simulink model "ptest3sim2"  (Simulink 6.3)
settings: Solver=FixedStepDiscrete  SolverMode=SingleTasking  StartTime=0.0  StopTime=999999  MaxStep=10  RelTol=1e-3  AbsTol=1e-6
settings Model: Creator=munlock -all d:\work\myr12\toolbox\fuzzy\fuzzy\mfedit.m  LastModifiedBy=mbharadw  ExtModeTrigMode=oneshot  ExtModeArmWhenConnect=off  StrictBusMsg=None
settings DataIOCC: LimitDataPoints=off  SaveOutput=off  SaveTime=off
settings OptimizationCC: BooleanDataType=off
settings DebuggingCC: SolverPrmCheckMsg=none
settings HardwareCC: TargetUnknown=on
settings RTWCC: TemplateMakefile=grt_vc.tmf

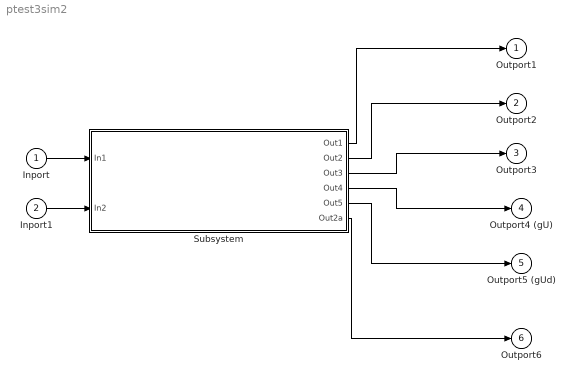
== system ptest3sim2 ==
  Inport : Inport  PortDimensions=1
  Inport1 : Inport  Port=2  PortDimensions=1
  Subsystem : Subsystem  mask{yd_init=, y_init=, ud_init=, u_init=, mint=, maxt=, minp=, maxp=, Ts=, S1=, Nu=, Normalize=, Nj=, Ni=, LW2_1=, LW1_2=, IW_gU=, IW=, B2=, B1=}
  Outport1 : Outport
  Outport2 : Outport  Port=2
  Outport3 : Outport  Port=3
  Outport4 (gU) : Outport  Port=4
  Outport5 (gUd) : Outport  Port=5
  Outport6 : Outport  Port=6
  wires:
  Subsystem/2(Out2) -> Outport2/1
  Subsystem/1(Out1) -> Outport1/1
  Subsystem/3(Out3) -> Outport3/1
  Inport1/1 -> Subsystem/2(In2)
  Subsystem/5(Out5) -> Outport5 (gUd)/1
  Inport/1 -> Subsystem/1(In1)
  Subsystem/4(Out4) -> Outport4 (gU)/1
  Subsystem/6(Out2a) -> Outport6/1

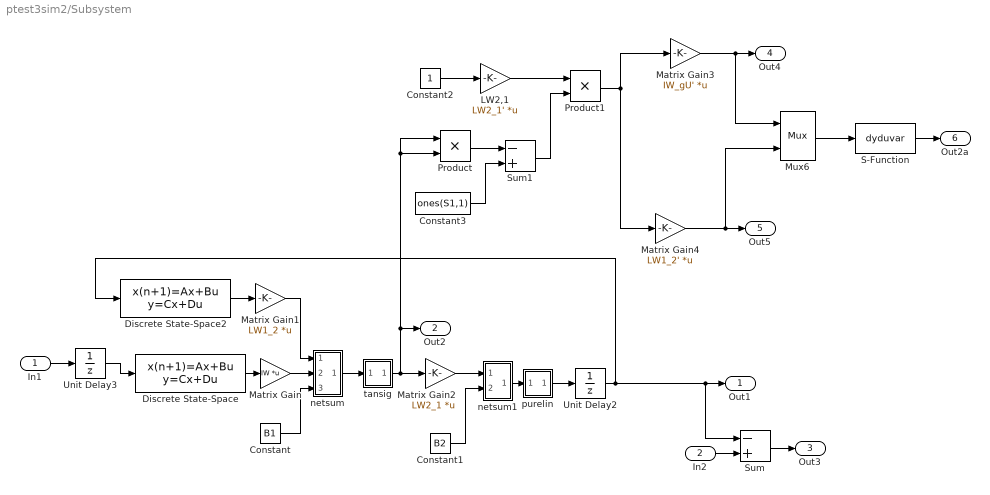
== system ptest3sim2/Subsystem ==
  In1 : Inport
  In2 : Inport  Port=2
  Constant : Constant  Value=B1
  Constant1 : Constant  Value=B2
  Constant2 : Constant
  Constant3 : Constant  Value=ones(S1,1)
  Discrete State-Space : DiscreteStateSpace  A=[0 zeros(1,Ni-2);eye(Ni-2,Ni-1)]  B=[zeros(double(Ni==1));eye(Ni-1,1)]  C=[0 zeros(1,Ni-2);eye(Ni-1,Ni-1)]  D=eye(Ni,1)  X0=ud_init  SampleTime=Ts
  Discrete State-Space2 : DiscreteStateSpace  A=[0 zeros(1,Nj-2);eye(Nj-2,Nj-1)]  B=[zeros(double(Nj==1));eye(Nj-1,1)]  C=[0 zeros(1,Nj-2);eye(Nj-1,Nj-1)]  D=eye(Nj,1)  X0=yd_init  SampleTime=Ts
  LW2,1 : Gain  Gain=LW2_1'  Multiplication=Matrix(K*u)  SaturateOnIntegerOverflow=on
  Matrix Gain : Gain  Gain=IW  Multiplication=Matrix(K*u)  SaturateOnIntegerOverflow=on
  Matrix Gain1 : Gain  Gain=LW1_2  Multiplication=Matrix(K*u)  SaturateOnIntegerOverflow=on
  Matrix Gain2 : Gain  Gain=LW2_1  Multiplication=Matrix(K*u)  SaturateOnIntegerOverflow=on
  Matrix Gain3 : Gain  Gain=IW_gU'  Multiplication=Matrix(K*u)  SaturateOnIntegerOverflow=on
  Matrix Gain4 : Gain  Gain=LW1_2'  Multiplication=Matrix(K*u)  SaturateOnIntegerOverflow=on
  Mux6 : Mux  Inputs=2
  Product : Product  SaturateOnIntegerOverflow=on  RndMeth=Zero  InputSameDT=on
  Product1 : Product  SaturateOnIntegerOverflow=on  RndMeth=Zero  InputSameDT=on
  S-Function : S-Function  FunctionName=dyduvar  Parameters=Nu,Ni,Nj,Ts,minp,maxp,mint,maxt,Normalize
  Sum : Sum  Inputs=-+  SaturateOnIntegerOverflow=on  InputSameDT=on
  Sum1 : Sum  Inputs=-+  SaturateOnIntegerOverflow=on  InputSameDT=on
  Unit Delay2 : UnitDelay  X0=y_init  SampleTime=Ts
  Unit Delay3 : UnitDelay  X0=u_init  SampleTime=Ts
  netsum : Subsystem
      mask Display: disp('+')
  netsum1 : Subsystem
      mask Display: disp('+')
  purelin : Subsystem
      mask Display: plot([-1 1],[0 0],[-1 1],[-1 1])
  tansig : Subsystem
      mask Display: plot([-1 1],[0 0],[-1 -.9 -.8 -.7 -.6 -.5 -.4 -.3 -.2 -.1 0 .1 .2 .3 .4 .5 .6 .7 .8 .9 1],2./(1+exp(-8*[-1 -.9 -.8 -.7 -.6 -.5 -.4 -.3 -.2 -.1 0 .1 .2 .3 .4 .5 .6 .7 .8 .9 1]))-1)
  Out1 : Outport
  Out2 : Outport  Port=2
  Out3 : Outport  Port=3
  Out4 : Outport  Port=4
  Out5 : Outport  Port=5
  Out2a : Outport  Port=6
  wires:
  LW2,1/1 -> Product1/1
  Product1/1 -> Matrix Gain4/1, Matrix Gain3/1
  Constant2/1 -> LW2,1/1
  Product/1 -> Sum1/1
  Constant3/1 -> Sum1/2
  Sum1/1 -> Product1/2
  netsum1/1(Out1) -> purelin/1(n)
  Constant1/1 -> netsum1/2(In2)
  Matrix Gain2/1 -> netsum1/1(In1)
  Constant/1 -> netsum/3(In3)
  Matrix Gain1/1 -> netsum/1(In1)
  Discrete State-Space2/1 -> Matrix Gain1/1
  Matrix Gain/1 -> netsum/2(In2)
  tansig/1(a) -> Product/1, Product/2, Out2/1, Matrix Gain2/1
  purelin/1(a) -> Unit Delay2/1
  Unit Delay2/1 -> Discrete State-Space2/1, Sum/1, Out1/1
  Discrete State-Space/1 -> Matrix Gain/1
  Matrix Gain4/1 -> Mux6/2, Out5/1
  Mux6/1 -> S-Function/1
  Unit Delay3/1 -> Discrete State-Space/1
  Matrix Gain3/1 -> Mux6/1, Out4/1
  S-Function/1 -> Out2a/1
  In1/1 -> Unit Delay3/1
  Sum/1 -> Out3/1
  In2/1 -> Sum/2
  netsum/1(Out1) -> tansig/1(n)

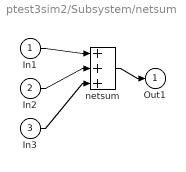
== system ptest3sim2/Subsystem/netsum ==
  In1 : Inport
  In2 : Inport  Port=2
  In3 : Inport  Port=3
  netsum : Sum  Inputs=3  SaturateOnIntegerOverflow=on  InputSameDT=on
  Out1 : Outport
  wires:
  In1/1 -> netsum/1
  In2/1 -> netsum/2
  In3/1 -> netsum/3
  netsum/1 -> Out1/1

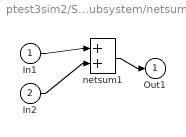
== system ptest3sim2/Subsystem/netsum1 ==
  In1 : Inport
  In2 : Inport  Port=2
  netsum1 : Sum  Inputs=2  SaturateOnIntegerOverflow=on  InputSameDT=on
  Out1 : Outport
  wires:
  In1/1 -> netsum1/1
  In2/1 -> netsum1/2
  netsum1/1 -> Out1/1

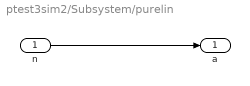
== system ptest3sim2/Subsystem/purelin ==
  n : Inport
  a : Outport
  wires:
  n/1 -> a/1

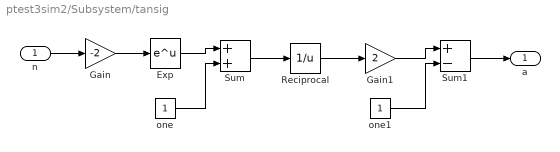
== system ptest3sim2/Subsystem/tansig ==
  n : Inport
  Exp : Math  SaturateOnIntegerOverflow=on
  Gain : Gain  Gain=-2  SaturateOnIntegerOverflow=on
  Gain1 : Gain  Gain=2  SaturateOnIntegerOverflow=on
  Reciprocal : Math  Operator=reciprocal  SaturateOnIntegerOverflow=on
  Sum : Sum  SaturateOnIntegerOverflow=on  InputSameDT=on
  Sum1 : Sum  Inputs=+-  SaturateOnIntegerOverflow=on  InputSameDT=on
  one : Constant
  one1 : Constant
  a : Outport
  wires:
  n/1 -> Gain/1
  Gain/1 -> Exp/1
  Exp/1 -> Sum/1
  one/1 -> Sum/2
  Sum/1 -> Reciprocal/1
  Reciprocal/1 -> Gain1/1
  Gain1/1 -> Sum1/1
  one1/1 -> Sum1/2
  Sum1/1 -> a/1
